simulink model "TCSC"  (R2022b)
settings: Solver=VariableStepAuto  StartTime=0.0  StopTime=.5  RelTol=1e-3
libraries: spsCurrentMeasurementLib x4, spsSeriesRLCBranchLib x4, dspsigops x2, spsThyristorLib x2, spsVoltageMeasurementLib x2, spsACVoltageSourceLib x1, simulink x1, sps_lib x1
settings Model: Creator=hp  LastModifiedBy=rishi kumar singh

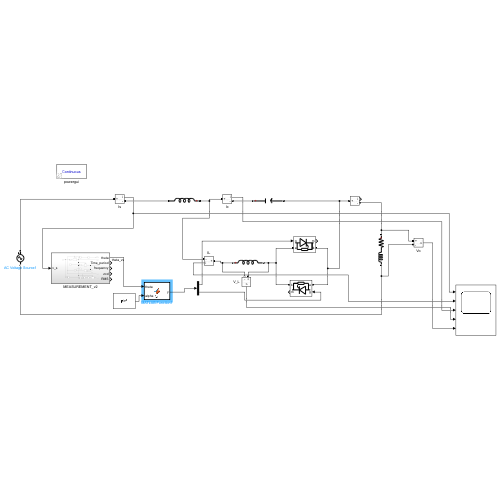
[thumbnail: Simulink's stored preview of the top-level diagram]
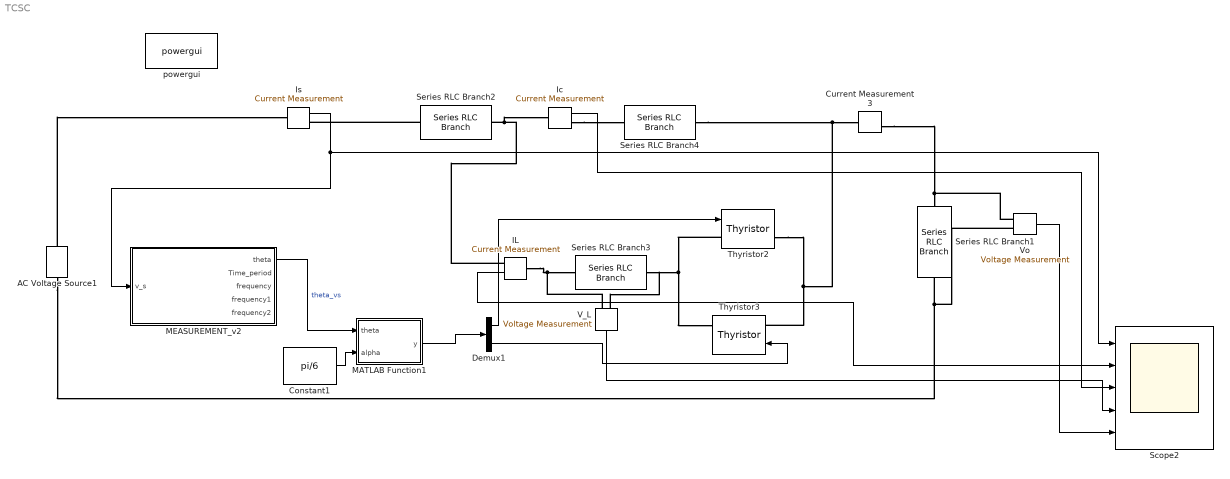
== system TCSC ==
  AC Voltage Source1 : spsACVoltageSourceLib/AC Voltage Source  Amplitude=20000*sqrt(2)  Phase=0  Frequency=50  SampleTime=0  Measurements=None  BusType=swing  Pref=10e3  Qref=0  Qmin=-inf  Qmax=+inf
  Constant1 : Constant  Value=pi/6
  Current Measurement3 : spsCurrentMeasurementLib/Current Measurement  PhasorSimulation=off  OutputType=Complex  PSBequivalent=0
  Demux1 : Demux  Outputs=2
  IL : spsCurrentMeasurementLib/Current Measurement  PhasorSimulation=off  OutputType=Complex  PSBequivalent=0
  Ic : spsCurrentMeasurementLib/Current Measurement  PhasorSimulation=off  OutputType=Complex  PSBequivalent=0
  Is : spsCurrentMeasurementLib/Current Measurement  PhasorSimulation=off  OutputType=Complex  PSBequivalent=0
  MATLAB Function1 : MATLAB Function  TreatAsAtomicUnit=on
  MEASUREMENT_v2 : Subsystem
  Scope2 : Scope  NumInputPorts=5
  Series RLC Branch1 : spsSeriesRLCBranchLib/Series RLC Branch  LConnTagsString=__new0  RConnTagsString=__new0  BranchType=RL  Resistance=20  Inductance=63.69e-3  SetiL0=off  InitialCurrent=0  Capacitance=1e-6  Setx0=off  InitialVoltage=0  Measurements=None
  Series RLC Branch2 : spsSeriesRLCBranchLib/Series RLC Branch  LConnTagsString=__new0  RConnTagsString=__new0  BranchType=L  Resistance=1  Inductance=31.8e-3  SetiL0=off  InitialCurrent=0  Capacitance=1e-6  Setx0=off  InitialVoltage=0  Measurements=None
  Series RLC Branch3 : spsSeriesRLCBranchLib/Series RLC Branch  LConnTagsString=__new0  RConnTagsString=__new0  BranchType=L  Resistance=1  Inductance=63.69e-3  SetiL0=off  InitialCurrent=0  Capacitance=1e-6  Setx0=off  InitialVoltage=0  Measurements=None
  Series RLC Branch4 : spsSeriesRLCBranchLib/Series RLC Branch  LConnTagsString=__new0  RConnTagsString=__new0  BranchType=C  Resistance=1  Inductance=63.69e-3  SetiL0=off  InitialCurrent=0  Capacitance=159.24e-6  Setx0=off  InitialVoltage=0  Measurements=None
  Thyristor2 : spsThyristorLib/Thyristor  Ron=0.001  Lon=0  Vf=0.8  IC=0  Rs=500  Cs=250e-9  Measurements=on
  Thyristor3 : spsThyristorLib/Thyristor  Ron=0.001  Lon=0  Vf=0.8  IC=0  Rs=500  Cs=250e-9  Measurements=on
  V_L : spsVoltageMeasurementLib/Voltage Measurement  PhasorSimulation=off  OutputType=Complex  PSBequivalent=0
  Vo : spsVoltageMeasurementLib/Voltage Measurement  PhasorSimulation=off  OutputType=Complex  PSBequivalent=0
  powergui : sps_lib/powergui  Priority=1  SimulationMode=Continuous  SampleTime=50e-6  frequency=60  Iterations=50  frequencyindice=50  Pbase=100e6  ErrMax=1e-4  UnitsV=kV  UnitsW=MW  buscounter=0  FunctionMessages=off  echomessages=off  EnableUseOfTLC=off  CurrentSourceSwitches=off  DisableSnubberDevices=off  DisableRonSwitches=off  DisableVfSwitches=off  DisplayEquations=off  AutomaticDiscreteSolvers=off  SolverType=Tustin/Backward Euler (TBE)  Interpol=off  ExternalGateDelay=off  methode=off  Ts=100  x0status=blocks  SPID=on  SwTol=0  HookPort=off  NonlinearTolerance=1e-4  nMaxIteration=100  ContinueOnMaxIteration=off  RestoreLinks=warning  ResistiveCurrentMeasurement=off  Frange=[0:2:500]  Ylog=off  Xlog=on  ShowGrid=off  save=off  variable=ZData  structure=0  ZoomFFT=off  StartTime=0.0  cycles=1  DisplayStyle=1  fundamental=60  FreqAxis=off  MaxFrequency=1000  frequencyindicesteady=1  RmsSteady=1  display=off
  wires:
  Constant1/1 -> MATLAB Function1/2(alpha)
  MEASUREMENT_v2/1(theta) -> MATLAB Function1/1(theta)  "theta_vs"
  MATLAB Function1/1(y) -> Demux1/1
  Is/1 -> MEASUREMENT_v2/1(v_s), Scope2/1
  Demux1/1 -> Thyristor2/1
  Demux1/2 -> Thyristor3/1
  IL/1 -> Scope2/2
  Ic/1 -> Scope2/3
  V_L/1 -> Scope2/4
  Vo/1 -> Scope2/5
  connections:
  AC Voltage Source1/LConn1 -- Vo/LConn2 -- Series RLC Branch1/RConn1
  Current Measurement3/RConn1 -- Vo/LConn1 -- Series RLC Branch1/LConn1
  AC Voltage Source1/RConn1 -- Is/LConn1
  Series RLC Branch2/RConn1 -- Is/RConn1
  Series RLC Branch2/LConn1 -- Ic/LConn1 -- IL/RConn1
  Thyristor2/RConn1 -- Thyristor3/LConn1 -- Current Measurement3/LConn1 -- Series RLC Branch4/RConn1
  Thyristor2/LConn1 -- V_L/LConn1 -- Series RLC Branch3/RConn1 -- Thyristor3/RConn1
  Ic/RConn1 -- Series RLC Branch4/LConn1
  IL/LConn1 -- V_L/LConn2 -- Series RLC Branch3/LConn1

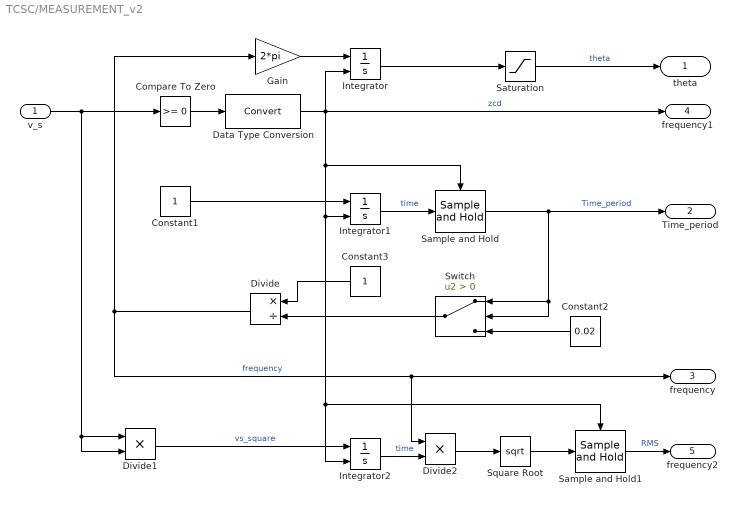
== system TCSC/MEASUREMENT_v2 ==
  v_s : Inport
  Compare To Zero : simulink/Logic and Bit Operations/Compare To Zero  relop=>=  OutDataTypeStr=boolean
  Constant1 : Constant
  Constant2 : Constant  Value=0.02
  Constant3 : Constant
  Data Type Conversion : DataTypeConversion  SaturateOnIntegerOverflow=off  RndMeth=Floor
  Divide : Product  Inputs=*/
  Divide1 : Product  Inputs=**
  Divide2 : Product  Inputs=**
  Gain : Gain  Gain=2*pi
  Integrator : Integrator  ExternalReset=rising
  Integrator1 : Integrator  ExternalReset=rising
  Integrator2 : Integrator  ExternalReset=rising
  Sample and Hold : dspsigops/Sample and Hold  trig=Rising edge  initCond=0  latchinput=on
  Sample and Hold1 : dspsigops/Sample and Hold  trig=Rising edge  initCond=0  latchinput=on
  Saturation : Saturate  UpperLimit=2*pi  LowerLimit=-2*pi
  Square Root : Sqrt
  Switch : Switch  Criteria=u2 > Threshold  SaturateOnIntegerOverflow=off  InputSameDT=off
  theta : Outport
  Time_period : Outport  Port=2
  frequency : Outport  Port=3
  frequency1 : Outport  Port=4
  frequency2 : Outport  Port=5
  wires:
  Compare To Zero/1 -> Data Type Conversion/1
  Constant3/1 -> Divide/1
  Integrator/1 -> Saturation/1
  Divide/1 -> Gain/1, Divide2/1, frequency/1  "frequency"
  Data Type Conversion/1 -> Integrator1/2, Sample and Hold1/Trigger, Integrator2/2, Sample and Hold/Trigger, frequency1/1, Integrator/2  "zcd"
  Gain/1 -> Integrator/1
  Sample and Hold/1 -> Time_period/1, Switch/2, Switch/1  "Time_period"
  Constant2/1 -> Switch/3
  Constant1/1 -> Integrator1/1
  Integrator1/1 -> Sample and Hold/1  "time"
  Switch/1 -> Divide/2
  v_s/1 -> Divide1/2, Divide1/1, Compare To Zero/1
  Divide1/1 -> Integrator2/1  "vs_square"
  Integrator2/1 -> Divide2/2  "time"
  Divide2/1 -> Square Root/1
  Square Root/1 -> Sample and Hold1/1
  Sample and Hold1/1 -> frequency2/1  "RMS"
  Saturation/1 -> theta/1  "theta"

== matlab function TCSC/MATLAB Function1 ==
  data: theta input; y output; alpha input
function y = fcn(theta,alpha)
gi=[0 0];
if(alpha == 0)
    gi=[0 0];
else
if(theta>= alpha && theta< pi/2)
    gi=[0 1];
end
if(theta>=pi+alpha && theta <3*pi/2)
    gi=[1 0];
end
end
y=gi;
